simulink library "sm_motor_grader_lib"  (R2026a)
settings: Solver=VariableStepAuto
undefined symbols (not defined in the file): activeTestCmds, Art, Center, Circle, Driver, HMPST, LiftL, LiftR, LnL, LnR, Loads, Maneuver, motGradParams, Pin, RFL, RFR, RRL, RRR, SceneData, Side, Sphere, StrL, StrR, Tilt, X, Y, Z
libraries: sm_lib x219, nesl_utility x134, fl_lib x53, $bdroot x24, cvt_powertrain_lib x6, simulink_extras x5, grid_element x4, simulink x3, cvt_powertrain_lib_vnts x3, Driver_Long_Lat_Stanley x1, Maneuver_Get_Pose x1, SignalEditorBlockLib x1
(part 13 of 13)

== system sm_motor_grader_lib/LiftAssembly/Saddle L/Actuator/Shaft ==
  p : Inport
  Abs : Abs  ZeroCross=off  SaturateOnIntegerOverflow=off
  Cylindrical Lift L : sm_lib/Joints/Cylindrical Joint  JointMode=Normal  CompositeWrenchDir=FollowerOnBase  CompositeWrenchFrame=BaseFrame  SenseConstraintForce=off  SenseConstraintTorque=off  SenseTotalForce=off  SenseTotalTorque=off  RzPositionTargetSpecify=off  RzPositionTargetPriority=High  RzPositionTargetValue=0  RzPositionTargetValueUnits=deg  RzVelocityTargetSpecify=off  RzVelocityTargetPriority=High  RzVelocityTargetValue=0  RzVelocityTargetValueUnits=deg/s  RzEquilibriumPosition=0  RzEquilibriumPositionUnits=deg  RzSpringStiffness=0  RzSpringStiffnessUnits=N*m/deg  RzDampingCoefficient=0  RzDampingCoefficientUnits=N*m/(deg/s)  RzLowerLimitSpecify=off  RzLowerLimitBound=-90  RzLowerLimitBoundUnits=deg  RzLowerLimitStiffness=1e4  RzLowerLimitStiffnessUnits=N*m/deg  RzLowerLimitDamping=10  RzLowerLimitDampingUnits=N*m/(deg/s)  RzLowerLimitTransitionRegionWidth=0.1  RzLowerLimitTransitionRegionWidthUnits=deg  RzUpperLimitSpecify=off  RzUpperLimitBound=90  RzUpperLimitBoundUnits=deg  RzUpperLimitStiffness=1e4  RzUpperLimitStiffnessUnits=N*m/deg  RzUpperLimitDamping=10  RzUpperLimitDampingUnits=N*m/(deg/s)  RzUpperLimitTransitionRegionWidth=0.1  RzUpperLimitTransitionRegionWidthUnits=deg  RzTorqueActuationMode=NoTorque  RzMotionActuationMode=ComputedMotion  RzSensePosition=off  RzSenseVelocity=off  RzSenseAcceleration=off  RzSenseTorqueForce=off  RzSenseLowerLimitTorqueForce=off  RzSenseUpperLimitTorqueForce=off  PzPositionTargetSpecify=on  PzPositionTargetPriority=High  PzPositionTargetValue=motGradParams.bladeLift.leftInitPos  PzPositionTargetValueUnits=m  PzVelocityTargetSpecify=off  PzVelocityTargetPriority=High  PzVelocityTargetValue=0  PzVelocityTargetValueUnits=m/s  PzEquilibriumPosition=0  PzEquilibriumPositionUnits=m  PzSpringStiffness=0  PzSpringStiffnessUnits=N/m  PzDampingCoefficient=0  PzDampingCoefficientUnits=N/(m/s)  PzLowerLimitSpecify=on  PzLowerLimitBound=0  PzLowerLimitBoundUnits=m  PzLowerLimitStiffness=1e6  PzLowerLimitStiffnessUnits=N/m  PzLowerLimitDamping=1e3  PzLowerLimitDampingUnits=N/(m/s)  PzLowerLimitTransitionRegionWidth=1e-4  PzLowerLimitTransitionRegionWidthUnits=m  PzUpperLimitSpecify=on  PzUpperLimitBound=motGradParams.bladeLift.stroke  PzUpperLimitBoundUnits=m  PzUpperLimitStiffness=1e6  PzUpperLimitStiffnessUnits=N/m  PzUpperLimitDamping=1e3  PzUpperLimitDampingUnits=N/(m/s)  PzUpperLimitTransitionRegionWidth=1e-4  PzUpperLimitTransitionRegionWidthUnits=m  PzTorqueActuationMode=InputTorque  PzMotionActuationMode=ComputedMotion  PzSensePosition=on  PzSenseVelocity=on  PzSenseAcceleration=off  PzSenseTorqueForce=on  PzSenseLowerLimitTorqueForce=off  PzSenseUpperLimitTorqueForce=off
  Mechanical Translational Reference : fl_lib/Mechanical/Translational Elements/Mechanical Translational Reference
  PS-Simulink Converter1 : nesl_utility/PS-Simulink Converter  PhysicalDomain=network_engine_domain  SubClassName=ps_output  LeftPortType=input  RightPortType=output  PseudoPeriodic=off  Frequencies=[]  VectorFormat=inherit  Unit=inherit  AffineConversion=off
  PS-Simulink Converter2 : nesl_utility/PS-Simulink Converter  PhysicalDomain=network_engine_domain  SubClassName=ps_output  LeftPortType=input  RightPortType=output  PseudoPeriodic=off  Frequencies=[]  VectorFormat=inherit  Unit=inherit  AffineConversion=off
  PS-Simulink Converter3 : nesl_utility/PS-Simulink Converter  PhysicalDomain=network_engine_domain  SubClassName=ps_output  LeftPortType=input  RightPortType=output  PseudoPeriodic=off  Frequencies=[]  VectorFormat=inherit  Unit=inherit  AffineConversion=off
  Product : Product
  Terminator : Terminator
  Translational Multibody Interface : fl_lib/Mechanical/Multibody Interfaces/Translational Multibody Interface
  R : PMIOPort  Side=Left
  B : PMIOPort  Port=2  Side=Left
  F : PMIOPort  Port=3  Side=Right
  Out Bus Element : Outport  PortName=m  Element=power
  Out Bus Element1 : Outport  PortName=m  Element=force
  Out Bus Element2 : Outport  PortName=m  Element=v
  Out Bus Element3 : Outport  PortName=m  Element=p
  wires:
  PS-Simulink Converter3/1 -> Out Bus Element3/1
  Product/1 -> Abs/1
  PS-Simulink Converter2/1 -> Out Bus Element2/1, Product/1
  Abs/1 -> Out Bus Element/1
  PS-Simulink Converter1/1 -> Out Bus Element1/1, Product/2
  p/1 -> Terminator/1
  connections:
  F/RConn1 -- Cylindrical Lift L/RConn1
  B/RConn1 -- Cylindrical Lift L/LConn1
  PS-Simulink Converter3/LConn1 -- Cylindrical Lift L/RConn2
  Translational Multibody Interface/LConn1 -- Cylindrical Lift L/LConn2
  Cylindrical Lift L/RConn3 -- PS-Simulink Converter2/LConn1 -- Translational Multibody Interface/RConn1
  Translational Multibody Interface/LConn2 -- Mechanical Translational Reference/LConn1
  R/RConn1 -- Translational Multibody Interface/RConn2
  PS-Simulink Converter1/LConn1 -- Cylindrical Lift L/RConn4

== system sm_motor_grader_lib/LiftAssembly/Saddle R/Actuator/Position ==
  p : Inport
  Abs : Abs  ZeroCross=off  SaturateOnIntegerOverflow=off
  Cylindrical Lift R : sm_lib/Joints/Cylindrical Joint  JointMode=Normal  CompositeWrenchDir=FollowerOnBase  CompositeWrenchFrame=BaseFrame  SenseConstraintForce=off  SenseConstraintTorque=off  SenseTotalForce=off  SenseTotalTorque=off  RzPositionTargetSpecify=off  RzPositionTargetPriority=High  RzPositionTargetValue=0  RzPositionTargetValueUnits=deg  RzVelocityTargetSpecify=off  RzVelocityTargetPriority=High  RzVelocityTargetValue=0  RzVelocityTargetValueUnits=deg/s  RzEquilibriumPosition=0  RzEquilibriumPositionUnits=deg  RzSpringStiffness=0  RzSpringStiffnessUnits=N*m/deg  RzDampingCoefficient=0  RzDampingCoefficientUnits=N*m/(deg/s)  RzLowerLimitSpecify=off  RzLowerLimitBound=-90  RzLowerLimitBoundUnits=deg  RzLowerLimitStiffness=1e4  RzLowerLimitStiffnessUnits=N*m/deg  RzLowerLimitDamping=10  RzLowerLimitDampingUnits=N*m/(deg/s)  RzLowerLimitTransitionRegionWidth=0.1  RzLowerLimitTransitionRegionWidthUnits=deg  RzUpperLimitSpecify=off  RzUpperLimitBound=90  RzUpperLimitBoundUnits=deg  RzUpperLimitStiffness=1e4  RzUpperLimitStiffnessUnits=N*m/deg  RzUpperLimitDamping=10  RzUpperLimitDampingUnits=N*m/(deg/s)  RzUpperLimitTransitionRegionWidth=0.1  RzUpperLimitTransitionRegionWidthUnits=deg  RzTorqueActuationMode=NoTorque  RzMotionActuationMode=ComputedMotion  RzSensePosition=off  RzSenseVelocity=off  RzSenseAcceleration=off  RzSenseTorqueForce=off  RzSenseLowerLimitTorqueForce=off  RzSenseUpperLimitTorqueForce=off  PzPositionTargetSpecify=on  PzPositionTargetPriority=High  PzPositionTargetValue=motGradParams.bladeLift.rightInitPos  PzPositionTargetValueUnits=m  PzVelocityTargetSpecify=off  PzVelocityTargetPriority=High  PzVelocityTargetValue=0  PzVelocityTargetValueUnits=m/s  PzEquilibriumPosition=0  PzEquilibriumPositionUnits=m  PzSpringStiffness=0  PzSpringStiffnessUnits=N/m  PzDampingCoefficient=0  PzDampingCoefficientUnits=N/(m/s)  PzLowerLimitSpecify=on  PzLowerLimitBound=0  PzLowerLimitBoundUnits=m  PzLowerLimitStiffness=1e6  PzLowerLimitStiffnessUnits=N/m  PzLowerLimitDamping=1e3  PzLowerLimitDampingUnits=N/(m/s)  PzLowerLimitTransitionRegionWidth=1e-4  PzLowerLimitTransitionRegionWidthUnits=m  PzUpperLimitSpecify=on  PzUpperLimitBound=motGradParams.bladeLift.stroke  PzUpperLimitBoundUnits=m  PzUpperLimitStiffness=1e6  PzUpperLimitStiffnessUnits=N/m  PzUpperLimitDamping=1e3  PzUpperLimitDampingUnits=N/(m/s)  PzUpperLimitTransitionRegionWidth=1e-4  PzUpperLimitTransitionRegionWidthUnits=m  PzTorqueActuationMode=ComputedTorque  PzMotionActuationMode=InputMotion  PzSensePosition=on  PzSenseVelocity=on  PzSenseAcceleration=off  PzSenseTorqueForce=on  PzSenseLowerLimitTorqueForce=off  PzSenseUpperLimitTorqueForce=off
  PS-Simulink Converter : nesl_utility/PS-Simulink Converter  PhysicalDomain=network_engine_domain  SubClassName=ps_output  LeftPortType=input  RightPortType=output  PseudoPeriodic=off  Frequencies=[]  VectorFormat=inherit  Unit=inherit  AffineConversion=off
  PS-Simulink Converter1 : nesl_utility/PS-Simulink Converter  PhysicalDomain=network_engine_domain  SubClassName=ps_output  LeftPortType=input  RightPortType=output  PseudoPeriodic=off  Frequencies=[]  VectorFormat=inherit  Unit=inherit  AffineConversion=off
  PS-Simulink Converter2 : nesl_utility/PS-Simulink Converter  PhysicalDomain=network_engine_domain  SubClassName=ps_output  LeftPortType=input  RightPortType=output  PseudoPeriodic=off  Frequencies=[]  VectorFormat=inherit  Unit=inherit  AffineConversion=off
  Product : Product
  Simulink-PS Converter : nesl_utility/Simulink-PS Converter  PhysicalDomain=network_engine_domain  SubClassName=ps_input  LeftPortType=input  RightPortType=output  PseudoPeriodic=off  Frequencies=[]  NoiseDistribution=none  NoiseParameters=[]  Unit=m  AffineConversion=off  FilteringAndDerivatives=filter  SimscapeFilterOrder=2  InputFilterTimeConstant=0.001  UdotUserProvided=0
  R : PMIOPort  Side=Left
  B : PMIOPort  Port=2  Side=Left
  F : PMIOPort  Port=3  Side=Right
  Out Bus Element : Outport  PortName=m  Element=power
  Out Bus Element1 : Outport  PortName=m  Element=force
  Out Bus Element2 : Outport  PortName=m  Element=v
  Out Bus Element3 : Outport  PortName=m  Element=p
  wires:
  p/1 -> Simulink-PS Converter/1
  PS-Simulink Converter2/1 -> Out Bus Element3/1
  Product/1 -> Abs/1
  PS-Simulink Converter1/1 -> Out Bus Element2/1, Product/1
  Abs/1 -> Out Bus Element/1
  PS-Simulink Converter/1 -> Out Bus Element1/1, Product/2
  connections:
  Cylindrical Lift R/LConn2 -- Simulink-PS Converter/RConn1
  B/RConn1 -- Cylindrical Lift R/LConn1
  F/RConn1 -- Cylindrical Lift R/RConn1
  Cylindrical Lift R/RConn2 -- PS-Simulink Converter2/LConn1
  Cylindrical Lift R/RConn3 -- PS-Simulink Converter1/LConn1
  Cylindrical Lift R/RConn4 -- PS-Simulink Converter/LConn1

== system sm_motor_grader_lib/LiftAssembly/Saddle R/Actuator/Shaft ==
  p : Inport
  Abs : Abs  ZeroCross=off  SaturateOnIntegerOverflow=off
  Cylindrical Lift R : sm_lib/Joints/Cylindrical Joint  JointMode=Normal  CompositeWrenchDir=FollowerOnBase  CompositeWrenchFrame=BaseFrame  SenseConstraintForce=off  SenseConstraintTorque=off  SenseTotalForce=off  SenseTotalTorque=off  RzPositionTargetSpecify=off  RzPositionTargetPriority=High  RzPositionTargetValue=0  RzPositionTargetValueUnits=deg  RzVelocityTargetSpecify=off  RzVelocityTargetPriority=High  RzVelocityTargetValue=0  RzVelocityTargetValueUnits=deg/s  RzEquilibriumPosition=0  RzEquilibriumPositionUnits=deg  RzSpringStiffness=0  RzSpringStiffnessUnits=N*m/deg  RzDampingCoefficient=0  RzDampingCoefficientUnits=N*m/(deg/s)  RzLowerLimitSpecify=off  RzLowerLimitBound=-90  RzLowerLimitBoundUnits=deg  RzLowerLimitStiffness=1e4  RzLowerLimitStiffnessUnits=N*m/deg  RzLowerLimitDamping=10  RzLowerLimitDampingUnits=N*m/(deg/s)  RzLowerLimitTransitionRegionWidth=0.1  RzLowerLimitTransitionRegionWidthUnits=deg  RzUpperLimitSpecify=off  RzUpperLimitBound=90  RzUpperLimitBoundUnits=deg  RzUpperLimitStiffness=1e4  RzUpperLimitStiffnessUnits=N*m/deg  RzUpperLimitDamping=10  RzUpperLimitDampingUnits=N*m/(deg/s)  RzUpperLimitTransitionRegionWidth=0.1  RzUpperLimitTransitionRegionWidthUnits=deg  RzTorqueActuationMode=NoTorque  RzMotionActuationMode=ComputedMotion  RzSensePosition=off  RzSenseVelocity=off  RzSenseAcceleration=off  RzSenseTorqueForce=off  RzSenseLowerLimitTorqueForce=off  RzSenseUpperLimitTorqueForce=off  PzPositionTargetSpecify=on  PzPositionTargetPriority=High  PzPositionTargetValue=motGradParams.bladeLift.rightInitPos  PzPositionTargetValueUnits=m  PzVelocityTargetSpecify=off  PzVelocityTargetPriority=High  PzVelocityTargetValue=0  PzVelocityTargetValueUnits=m/s  PzEquilibriumPosition=0  PzEquilibriumPositionUnits=m  PzSpringStiffness=0  PzSpringStiffnessUnits=N/m  PzDampingCoefficient=0  PzDampingCoefficientUnits=N/(m/s)  PzLowerLimitSpecify=on  PzLowerLimitBound=0  PzLowerLimitBoundUnits=m  PzLowerLimitStiffness=1e6  PzLowerLimitStiffnessUnits=N/m  PzLowerLimitDamping=1e3  PzLowerLimitDampingUnits=N/(m/s)  PzLowerLimitTransitionRegionWidth=1e-4  PzLowerLimitTransitionRegionWidthUnits=m  PzUpperLimitSpecify=on  PzUpperLimitBound=motGradParams.bladeLift.stroke  PzUpperLimitBoundUnits=m  PzUpperLimitStiffness=1e6  PzUpperLimitStiffnessUnits=N/m  PzUpperLimitDamping=1e3  PzUpperLimitDampingUnits=N/(m/s)  PzUpperLimitTransitionRegionWidth=1e-4  PzUpperLimitTransitionRegionWidthUnits=m  PzTorqueActuationMode=InputTorque  PzMotionActuationMode=ComputedMotion  PzSensePosition=on  PzSenseVelocity=on  PzSenseAcceleration=off  PzSenseTorqueForce=on  PzSenseLowerLimitTorqueForce=off  PzSenseUpperLimitTorqueForce=off
  Mechanical Translational Reference : fl_lib/Mechanical/Translational Elements/Mechanical Translational Reference
  PS-Simulink Converter1 : nesl_utility/PS-Simulink Converter  PhysicalDomain=network_engine_domain  SubClassName=ps_output  LeftPortType=input  RightPortType=output  PseudoPeriodic=off  Frequencies=[]  VectorFormat=inherit  Unit=inherit  AffineConversion=off
  PS-Simulink Converter2 : nesl_utility/PS-Simulink Converter  PhysicalDomain=network_engine_domain  SubClassName=ps_output  LeftPortType=input  RightPortType=output  PseudoPeriodic=off  Frequencies=[]  VectorFormat=inherit  Unit=inherit  AffineConversion=off
  PS-Simulink Converter3 : nesl_utility/PS-Simulink Converter  PhysicalDomain=network_engine_domain  SubClassName=ps_output  LeftPortType=input  RightPortType=output  PseudoPeriodic=off  Frequencies=[]  VectorFormat=inherit  Unit=inherit  AffineConversion=off
  Product : Product
  Terminator : Terminator
  Translational Multibody Interface : fl_lib/Mechanical/Multibody Interfaces/Translational Multibody Interface
  R : PMIOPort  Side=Left
  B : PMIOPort  Port=2  Side=Left
  F : PMIOPort  Port=3  Side=Right
  Out Bus Element : Outport  PortName=m  Element=power
  Out Bus Element1 : Outport  PortName=m  Element=force
  Out Bus Element2 : Outport  PortName=m  Element=v
  Out Bus Element3 : Outport  PortName=m  Element=p
  wires:
  Abs/1 -> Out Bus Element/1
  PS-Simulink Converter1/1 -> Out Bus Element1/1, Product/2
  PS-Simulink Converter2/1 -> Out Bus Element2/1, Product/1
  Product/1 -> Abs/1
  p/1 -> Terminator/1
  PS-Simulink Converter3/1 -> Out Bus Element3/1
  connections:
  F/RConn1 -- Cylindrical Lift R/RConn1
  B/RConn1 -- Cylindrical Lift R/LConn1
  Translational Multibody Interface/LConn1 -- Cylindrical Lift R/LConn2
  Translational Multibody Interface/LConn2 -- Mechanical Translational Reference/LConn1
  R/RConn1 -- Translational Multibody Interface/RConn2
  Cylindrical Lift R/RConn2 -- PS-Simulink Converter3/LConn1
  Cylindrical Lift R/RConn3 -- Translational Multibody Interface/RConn1 -- PS-Simulink Converter2/LConn1
  Cylindrical Lift R/RConn4 -- PS-Simulink Converter1/LConn1

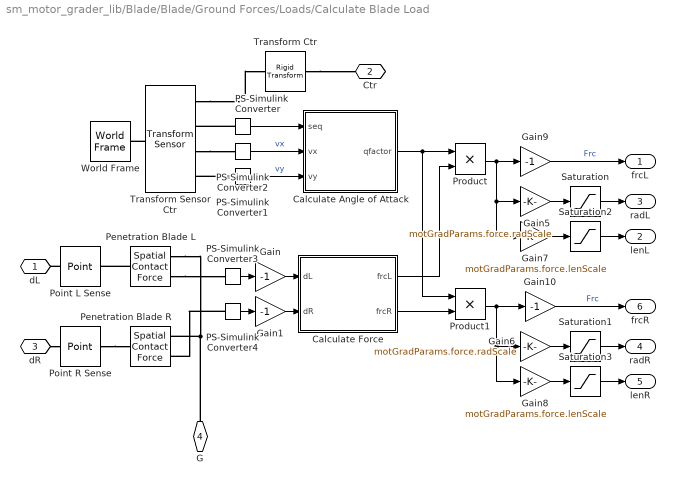
== system sm_motor_grader_lib/Blade/Blade/Ground Forces/Loads/Calculate Blade Load ==
  Calculate Angle of Attack : Subsystem
  Calculate Force : Subsystem
  Gain{,1,9..10} (4 alike) : Gain  Gain=-1
  Gain5 : Gain  Gain=motGradParams.force.radScale
  Gain6 : Gain  Gain=motGradParams.force.radScale
  Gain7 : Gain  Gain=motGradParams.force.lenScale
  Gain8 : Gain  Gain=motGradParams.force.lenScale
  PS-Simulink Converter : nesl_utility/PS-Simulink Converter  PhysicalDomain=network_engine_domain  SubClassName=ps_output  LeftPortType=input  RightPortType=output  PseudoPeriodic=off  Frequencies=[]  VectorFormat=inherit  Unit=rad  AffineConversion=off
  PS-Simulink Converter{1..4} (4 alike) : nesl_utility/PS-Simulink Converter  PhysicalDomain=network_engine_domain  SubClassName=ps_output  LeftPortType=input  RightPortType=output  PseudoPeriodic=off  Frequencies=[]  VectorFormat=inherit  Unit=inherit  AffineConversion=off
  Penetration Blade L : sm_lib/Forces and Torques/Spatial Contact Force  SenseSeparationDistance=off  NormalForceType=SmoothSpringDamper  NormalStiffness=0  NormalStiffnessUnits=N/m  NormalDamping=0  NormalDampingUnits=N/(m/s)  NormalTransitionRegionWidth=10  NormalTransitionRegionWidthUnits=m  FrictionType=SmoothStickSlip  CoefficientOfStaticFriction=0  CoefficientOfDynamicFriction=0  FrictionalCriticalVelocity=10  FrictionalCriticalVelocityUnits=m/s  SenseContactSignal=off  SensePenetrationDepth=on  SenseNormalVelocity=off  SenseTangentialVelocity=off  SensingForceTorqueDirection=BaseOnFollower  SensingForceTorqueResolutionFrame=ContactFrame  SenseNormalForce=off  SenseNormalForceMagnitude=off  SenseNormalTorque=off  SenseFrictionalForce=off  SenseFrictionalForceMagnitude=off  SenseFrictionalTorque=off  SenseTotalForce=off  SenseTotalTorque=off  SenseContactBaseRotation=off  SenseContactBaseTranslation=off  SenseContactFollowerRotation=off  SenseContactFollowerTranslation=off  ZeroCrossDetectContactStartAndEnd=off
  Penetration Blade R : sm_lib/Forces and Torques/Spatial Contact Force  SenseSeparationDistance=off  NormalForceType=SmoothSpringDamper  NormalStiffness=0  NormalStiffnessUnits=N/m  NormalDamping=0  NormalDampingUnits=N/(m/s)  NormalTransitionRegionWidth=10  NormalTransitionRegionWidthUnits=m  FrictionType=SmoothStickSlip  CoefficientOfStaticFriction=0  CoefficientOfDynamicFriction=0  FrictionalCriticalVelocity=10  FrictionalCriticalVelocityUnits=m/s  SenseContactSignal=off  SensePenetrationDepth=on  SenseNormalVelocity=off  SenseTangentialVelocity=off  SensingForceTorqueDirection=BaseOnFollower  SensingForceTorqueResolutionFrame=ContactFrame  SenseNormalForce=off  SenseNormalForceMagnitude=off  SenseNormalTorque=off  SenseFrictionalForce=off  SenseFrictionalForceMagnitude=off  SenseFrictionalTorque=off  SenseTotalForce=off  SenseTotalTorque=off  SenseContactBaseRotation=off  SenseContactBaseTranslation=off  SenseContactFollowerRotation=off  SenseContactFollowerTranslation=off  ZeroCrossDetectContactStartAndEnd=off
  Point L Sense : sm_lib/Curves and Surfaces/Point  GraphicType=None  MarkerShape=Sphere  MarkerSize=10  GraphicVisPropType=SimpleVisualProperties  GraphicDiffuseColor=[0.5 0.5 0.5]  GraphicOpacity=1  GraphicSpecularColor=[0.5 0.5 0.5 1.0]  GraphicAmbientColor=[0.15 0.15 0.15 1.0]  GraphicEmissiveColor=[0.0 0.0 0.0 1.0]  GraphicShininess=75
  Point R Sense : sm_lib/Curves and Surfaces/Point  GraphicType=None  MarkerShape=Sphere  MarkerSize=10  GraphicVisPropType=SimpleVisualProperties  GraphicDiffuseColor=[0.5 0.5 0.5]  GraphicOpacity=1  GraphicSpecularColor=[0.5 0.5 0.5 1.0]  GraphicAmbientColor=[0.15 0.15 0.15 1.0]  GraphicEmissiveColor=[0.0 0.0 0.0 1.0]  GraphicShininess=75
  Product : Product
  Product1 : Product
  Saturation : Saturate  UpperLimit=motGradParams.force.cylRadMax  LowerLimit=0  ZeroCross=off
  Saturation1 : Saturate  UpperLimit=motGradParams.force.cylRadMax  LowerLimit=0  ZeroCross=off
  Saturation2 : Saturate  UpperLimit=motGradParams.force.cylLenMax  LowerLimit=0  ZeroCross=off
  Saturation3 : Saturate  UpperLimit=motGradParams.force.cylLenMax  LowerLimit=0  ZeroCross=off
  Transform Sensor Ctr : sm_lib/Frames and Transforms/Transform Sensor  MeasurementFrame=World  RotationSequence=ZYX  SenseAngle=off  SenseAxis=off  SenseQ=off  SenseR=off  SenseRotationSequence=on  SenseOmegaX=off  SenseOmegaY=off  SenseOmegaZ=off  SenseOmega=off  SenseQDot=off  SenseRDot=off  SenseRotationSequenceDot=off  SenseAlphaX=off  SenseAlphaY=off  SenseAlphaZ=off  SenseAlpha=off  SenseQDDot=off  SenseRDDot=off  SenseX=off  SenseY=off  SenseZ=off  SenseXYZ=off  SenseRad=off  SenseAzim=off  SenseDist=off  SenseInc=off  SenseXDot=on  SenseYDot=on  SenseZDot=off  SenseXYZDot=off  SenseRadDot=off  SenseAzimDot=off  SenseDistDot=off  SenseIncDot=off  SenseXDDot=off  SenseYDDot=off  SenseZDDot=off  SenseXYZDDot=off  SenseRadDDot=off  SenseAzimDDot=off  SenseDistDDot=off  SenseIncDDot=off
  Transform Ctr : sm_lib/Frames and Transforms/Rigid Transform  RotationMethod=StandardAxis  FollAlignAxisA=+X  BaseAlignAxisA=+Y  FollAlignAxisB=+Y  BaseAlignAxisB=+Z  RotationStandardAxis=+Z  RotationAngle=90  RotationAngleUnits=deg  RotationArbitraryAxis=[0 0 1]  RotationSequenceAxes=FollowerAxes  RotationSequence=XYX  RotationSequenceAngles=[0 0 0]  RotationSequenceAnglesUnits=deg  RotationMatrix=[1 0 0;0 1 0;0 0 1]  Quaternion=[1 0 0 0]  TranslationMethod=None  TranslationCartesianOffset=[0 0 0]  TranslationCartesianOffsetUnits=m  TranslationStandardAxis=+Z  TranslationStandardOffset=0  TranslationStandardOffsetUnits=m  TranslationROffset=0  TranslationROffsetUnits=m  TranslationThetaOffset=0  TranslationThetaOffsetUnits=deg  TranslationZOffset=0  TranslationZOffsetUnits=m
  World Frame : sm_lib/Frames and Transforms/World Frame
  dL : PMIOPort  Side=Left
  Ctr : PMIOPort  Port=2  Side=Left
  dR : PMIOPort  Port=3  Side=Left
  G : PMIOPort  Port=4  Side=Right
  frcL : Outport
  lenL : Outport  Port=2
  radL : Outport  Port=3
  radR : Outport  Port=4
  lenR : Outport  Port=5
  frcR : Outport  Port=6
  wires:
  PS-Simulink Converter4/1 -> Gain1/1
  Saturation/1 -> radL/1
  Saturation1/1 -> radR/1
  Saturation2/1 -> lenL/1
  Saturation3/1 -> lenR/1
  PS-Simulink Converter3/1 -> Gain/1
  Product/1 -> Gain9/1, Gain7/1, Gain5/1
  Product1/1 -> Gain10/1, Gain8/1, Gain6/1
  Gain5/1 -> Saturation/1
  Gain7/1 -> Saturation2/1
  Gain6/1 -> Saturation1/1
  Gain8/1 -> Saturation3/1
  Gain9/1 -> frcL/1  "Frc"
  Gain10/1 -> frcR/1  "Frc"
  Calculate Angle of Attack/1(qfactor) -> Product/1, Product1/1
  Calculate Force/1(frcL) -> Product/2
  Calculate Force/2(frcR) -> Product1/2
  PS-Simulink Converter/1 -> Calculate Angle of Attack/1(seq)
  PS-Simulink Converter2/1 -> Calculate Angle of Attack/2(vx)  "vx"
  PS-Simulink Converter1/1 -> Calculate Angle of Attack/3(vy)  "vy"
  Gain/1 -> Calculate Force/1(dL)
  Gain1/1 -> Calculate Force/2(dR)
  connections:
  Transform Ctr/LConn1 -- Ctr/RConn1
  Transform Sensor Ctr/RConn1 -- Transform Ctr/RConn1
  PS-Simulink Converter/LConn1 -- Transform Sensor Ctr/RConn2
  Transform Sensor Ctr/RConn3 -- PS-Simulink Converter2/LConn1
  PS-Simulink Converter1/LConn1 -- Transform Sensor Ctr/RConn4
  Transform Sensor Ctr/LConn1 -- World Frame/RConn1
  PS-Simulink Converter4/LConn1 -- Penetration Blade R/RConn2
  Penetration Blade L/RConn2 -- PS-Simulink Converter3/LConn1
  Penetration Blade L/LConn1 -- Point L Sense/RConn1
  Point L Sense/LConn1 -- dL/RConn1
  Point R Sense/RConn1 -- Penetration Blade R/LConn1
  dR/RConn1 -- Point R Sense/LConn1
  G/RConn1 -- Penetration Blade R/RConn1 -- Penetration Blade L/RConn1

== system sm_motor_grader_lib/Blade/Blade/Ground Forces/Loads/Calculate Blade Load/Calculate Angle of Attack ==
  note: Calculate relative angle between blade normal and vehicle forward velocity. Use relative angle to scale force on blade (max force when blade normal and vehicle velocity vector are aligned).
  seq : Inport
  vx : Inport  Port=2
  vy : Inport  Port=3
  Abs : Abs  ZeroCross=off  SaturateOnIntegerOverflow=off
  Atan2 : Trigonometry  Operator=atan2
  Constant : Constant  Value=90
  Gain : Gain  Gain=180/pi
  Gain1 : Gain  Gain=180/pi
  Gain2 : Gain  Gain=pi/180
  Mux : Mux  Inputs=3
  Product : Product
  Saturation : Saturate  UpperLimit=90  LowerLimit=0  ZeroCross=off
  Selector : Selector  InputPortWidth=3  IndexOptions=Index vector (dialog)  Indices=1  OutputSizes=1
  Sin : Trigonometry
  Sqrt : Sqrt
  Square : Math  Operator=square
  Square1 : Math  Operator=square
  Subtract : Sum  Inputs=+-
  Subtract1 : Sum  Inputs=+-
  Sum : Sum
  Terminator : Terminator
  Terminator1 : Terminator
  qfactor : Outport
  wires:
  Mux/1 -> Terminator1/1
  Gain1/1 -> Mux/2, Subtract/1  "qVeh"
  Subtract/1 -> Mux/3, Abs/1  "qNorm"
  Product/1 -> Terminator/1  "vRes"
  Gain/1 -> Mux/1, Subtract/2  "qBlade"
  Sin/1 -> qfactor/1, Product/1  "factor"
  Sqrt/1 -> Product/2
  Sum/1 -> Sqrt/1
  Square1/1 -> Sum/2
  Square/1 -> Sum/1
  vx/1 -> Square1/1, Atan2/2
  Gain2/1 -> Sin/1
  Saturation/1 -> Gain2/1
  seq/1 -> Selector/1
  Selector/1 -> Gain/1
  Constant/1 -> Subtract1/1
  Abs/1 -> Subtract1/2
  Atan2/1 -> Gain1/1
  Subtract1/1 -> Saturation/1
  vy/1 -> Square/1, Atan2/1

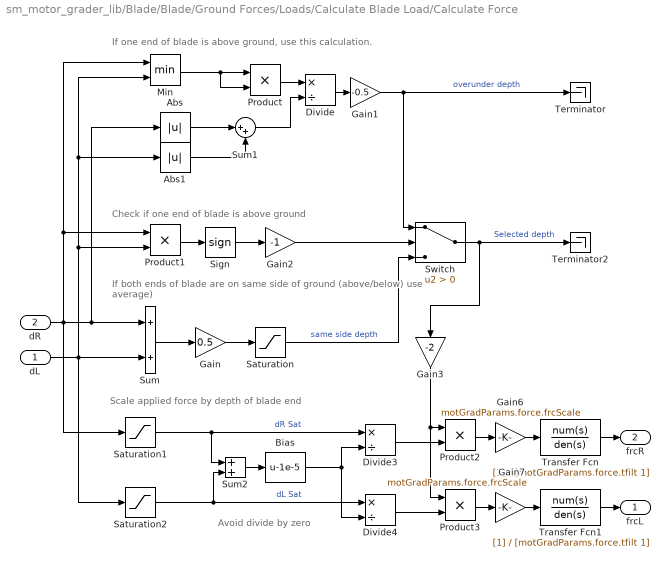
== system sm_motor_grader_lib/Blade/Blade/Ground Forces/Loads/Calculate Blade Load/Calculate Force ==
  note: Check if one end of blade is above ground
  note: If one end of blade is above ground, use this calculation.
  note: If both ends of blade are on same
      | side of ground (above/below) use average)
  note: Avoid divide by zero
  note: Scale applied force by depth of blade end
  dL : Inport
  dR : Inport  Port=2
  Abs : Abs  SaturateOnIntegerOverflow=off
  Abs1 : Abs  SaturateOnIntegerOverflow=off
  Bias : Bias  Bias=-1e-5  SaturateOnIntegerOverflow=off
  Divide : Product  Inputs=*/
  Divide3 : Product  Inputs=*/
  Divide4 : Product  Inputs=*/
  Gain : Gain  Gain=0.5
  Gain1 : Gain  Gain=-0.5
  Gain2 : Gain  Gain=-1
  Gain3 : Gain  Gain=-2
  Gain6 : Gain  Gain=motGradParams.force.frcScale
  Gain7 : Gain  Gain=motGradParams.force.frcScale
  Min : MinMax  Inputs=2
  Product{,1..3} (4 alike) : Product
  Saturation : Saturate  UpperLimit=0  LowerLimit=-inf  ZeroCross=off
  Saturation1 : Saturate  UpperLimit=0  LowerLimit=-inf  ZeroCross=off
  Saturation2 : Saturate  UpperLimit=0  LowerLimit=-inf  ZeroCross=off
  Sign : Signum
  Sum : Sum
  Sum1 : Sum  Inputs=|++
  Sum2 : Sum
  Switch : Switch  Criteria=u2 > Threshold  ZeroCross=off  SaturateOnIntegerOverflow=off  InputSameDT=off
  Terminator : Terminator
  Terminator2 : Terminator
  Transfer Fcn : TransferFcn  Denominator=[motGradParams.force.tfilt 1]
  Transfer Fcn1 : TransferFcn  Denominator=[motGradParams.force.tfilt 1]
  frcL : Outport
  frcR : Outport  Port=2
  wires:
  Product2/1 -> Gain6/1
  Product3/1 -> Gain7/1
  Divide4/1 -> Product3/2
  Divide3/1 -> Product2/2
  Bias/1 -> Divide3/2, Divide4/2
  Sum2/1 -> Bias/1
  Sum/1 -> Gain/1
  dR/1 -> Product1/1, Min/1, Abs/1, Sum/1, Saturation1/1
  dL/1 -> Abs1/1, Min/2, Product1/2, Sum/2, Saturation2/1
  Gain/1 -> Saturation/1
  Saturation/1 -> Switch/3  "same side depth"
  Min/1 -> Product/2, Product/1
  Abs/1 -> Sum1/1
  Abs1/1 -> Sum1/2
  Product/1 -> Divide/1
  Sum1/1 -> Divide/2
  Divide/1 -> Gain1/1
  Gain1/1 -> Switch/1, Terminator/1  "overunder depth"
  Product1/1 -> Sign/1
  Sign/1 -> Gain2/1
  Switch/1 -> Gain3/1, Terminator2/1  "Selected depth"
  Gain2/1 -> Switch/2
  Saturation1/1 -> Sum2/1, Divide3/1  "dR Sat"
  Saturation2/1 -> Sum2/2, Divide4/1  "dL Sat"
  Gain3/1 -> Product2/1, Product3/1
  Gain6/1 -> Transfer Fcn/1
  Gain7/1 -> Transfer Fcn1/1
  Transfer Fcn/1 -> frcR/1
  Transfer Fcn1/1 -> frcL/1

== matlab function sm_motor_grader_lib/LiftAssembly/LinkBar/ModeSelector ==
  data: engagedHole input; centerMode output; leftOneMode output; leftTwoMode output; leftThreeMode output; rightOneMode output; rightTwoMode output; rightThreeMode output
function [centerMode, leftOneMode, leftTwoMode, leftThreeMode, ...
    rightOneMode, rightTwoMode, rightThreeMode] = ModeSelector(engagedHole)

centerMode = 0;
leftOneMode = 0;
leftTwoMode = 0;
leftThreeMode = 0;
rightOneMode = 0;
rightTwoMode = 0;
rightThreeMode = 0;

if engagedHole == 0
    centerMode = 1;
elseif engagedHole == -1
    leftOneMode = 1;
elseif engagedHole == -2
    leftTwoMode = 1;
elseif engagedHole == -3
    leftThreeMode = 1;
elseif engagedHole == 1
    rightOneMode = 1;
elseif engagedHole == 2
    rightTwoMode = 1;
elseif engagedHole == 3
    rightThreeMode = 1;
end
